simulink model "TransFunct"  (Simulink 7.5)
settings: Solver=ode45  StartTime=0.0  StopTime=10.0  RelTol=1e-3
settings Model: Creator=My Laptop  LastModifiedBy=My Laptop

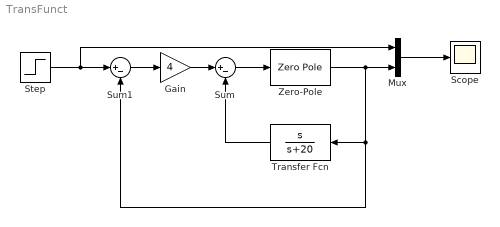
== system TransFunct ==
  Gain : Gain  Gain=4  ParameterDataType=fixdt(1, 16)  ParameterScaling=2^0  OutDataType=fixdt(1, 16)  OutScaling=2^0
  Mux : Mux  Inputs=2
  Scope : Scope
      settings: YMin=-1  YMax=140
  Step : Step  Time=0  SampleTime=0
  Sum : Sum  Inputs=|+-  OutDataType=fixdt(1, 16)  OutScaling=2^0
  Sum1 : Sum  Inputs=|+-  OutDataType=fixdt(1, 16)  OutScaling=2^0
  Transfer Fcn : TransferFcn  Numerator=[1 0]  Denominator=[1 20]
  Zero-Pole : ZeroPole  Zeros=[]  Poles=[0 -2]  Gain=[100]
  wires:
  Sum1/1 -> Gain/1
  Gain/1 -> Sum/1
  Sum/1 -> Zero-Pole/1
  Zero-Pole/1 -> Transfer Fcn/1, Sum1/2, Mux/2
  Transfer Fcn/1 -> Sum/2
  Step/1 -> Sum1/1, Mux/1
  Mux/1 -> Scope/1
